simulink model "hybrid_discharge_sc_bat"  (R2014b)
settings: Solver=ode23t  StartTime=0.0  StopTime=10  RelTol=1e-3
undefined symbols (not defined in the file or in its folder): Hydride, Metal, Nickel
libraries: powerlib x9, simulink x3, electricdrivelib x2
settings Model: Creator=Administrator  LastModifiedBy=Administrator

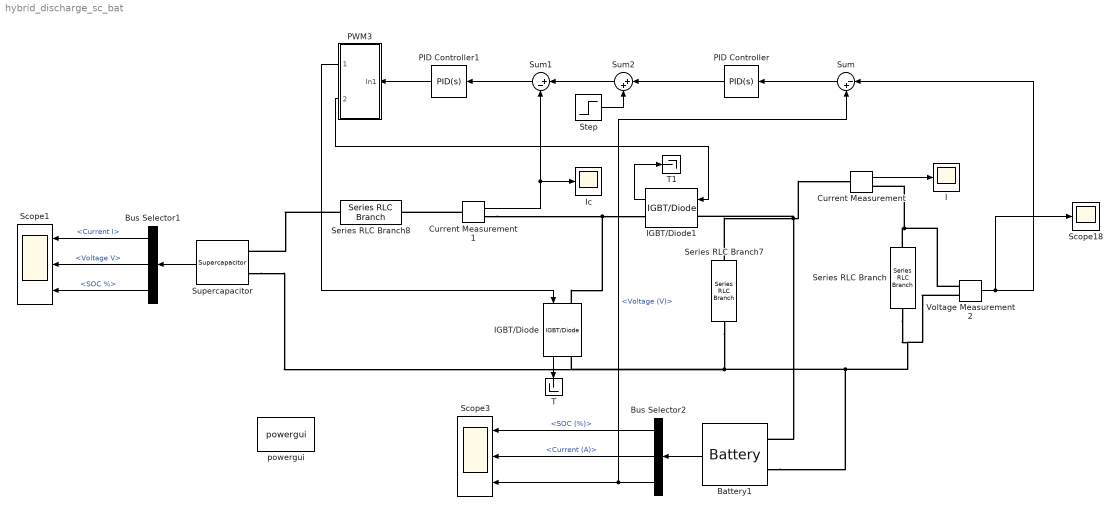
== system hybrid_discharge_sc_bat ==
  Battery1 : electricdrivelib/Extra Sources/Battery  BatType=Nickel-Metal-Hydride  ShowDetailedParameters=off  NomV=380  NomQ=100  SOC=80  PresetModel=on  MaxQ=107.6923  FullV=447.6271  Dis_rate=20  R=0.038  Normal_OP=96.1538  expZone="[412.2034            20]"  Dis_Char=off  current=[1.5 3]  Units=Ampere-hour  Batt_Tr=30
  Bus Selector1 : BusSelector  OutputSignals=Current I,Voltage V,SOC %
  Bus Selector2 : BusSelector  OutputSignals=SOC (%),Current (A),Voltage (V)
  Current Measurement : powerlib/Measurements/Current Measurement  PhasorSimulation=off  OutputType=Complex  PSBequivalent=0
  Current Measurement1 : powerlib/Measurements/Current Measurement  PhasorSimulation=off  OutputType=Complex  PSBequivalent=0
  I : Scope
      settings: YMin=750  YMax=1100  SaveName=ScopeData21  MaxDataPoints=5000000
  IGBT/Diode : powerlib/Power Electronics/IGBT//Diode  Ron=1e-3  Rs=1e5  Cs=inf  Measurements=on
  IGBT/Diode1 : powerlib/Power Electronics/IGBT//Diode  Ron=1e-3  Rs=1e5  Cs=inf  Measurements=on
  Ic : Scope
      settings: YMin=750  YMax=1100  SaveName=ScopeData3  MaxDataPoints=5000000
  PID Controller : simulink/Continuous/PID Controller  Controller=PID  TimeDomain=Continuous-time  SampleTime=-1  IntegratorMethod=Forward Euler  FilterMethod=Forward Euler  Form=Parallel  P=0.1  I=10  D=0  N=100  InitialConditionSource=internal  InitialConditionForIntegrator=0  InitialConditionForFilter=0  ExternalReset=none  LimitOutput=off  UpperSaturationLimit=inf  LowerSaturationLimit=-inf  LinearizeAsGain=on  AntiWindupMode=none  Kb=1  TrackingMode=off  Kt=1  PParamMin=[]  PParamMax=[]  IParamMin=[]  IParamMax=[]  DParamMin=[]  DParamMax=[]  NParamMin=[]  NParamMax=[]  KbParamMin=[]  KbParamMax=[]  KtParamMin=[]  KtParamMax=[]  POutMin=[]  POutMax=[]  IOutMin=[]  IOutMax=[]  DOutMin=[]  DOutMax=[]  NOutMin=[]  NOutMax=[]  KbOutMin=[]  KbOutMax=[]  KtOutMin=[]  KtOutMax=[]  IntegratorOutMin=[]  IntegratorOutMax=[]  FilterOutMin=[]  FilterOutMax=[]  SumOutMin=[]  SumOutMax=[]  SumI1OutMin=[]  SumI1OutMax=[]  SumI2OutMin=[]  SumI2OutMax=[]  SumI3OutMin=[]  SumI3OutMax=[]  SumDOutMin=[]  SumDOutMax=[]  SaturationOutMin=[]  SaturationOutMax=[]  IntegratorContinuousStateAttributes=''  IntegratorStateMustResolveToSignalObject=off  IntegratorRTWStateStorageClass=Auto  FilterContinuousStateAttributes=''  FilterStateMustResolveToSignalObject=off  FilterRTWStateStorageClass=Auto  DifferentiatorICPrevScaledInput=0  DifferentiatorOutMin=[]  DifferentiatorOutMax=[]  UseFilter=on
  PID Controller1 : simulink/Continuous/PID Controller  Controller=PID  TimeDomain=Continuous-time  SampleTime=-1  IntegratorMethod=Forward Euler  FilterMethod=Forward Euler  Form=Parallel  P=0.1  I=1  D=0  N=100  InitialConditionSource=internal  InitialConditionForIntegrator=0  InitialConditionForFilter=0  ExternalReset=none  LimitOutput=off  UpperSaturationLimit=inf  LowerSaturationLimit=-inf  LinearizeAsGain=on  AntiWindupMode=none  Kb=1  TrackingMode=off  Kt=1  PParamMin=[]  PParamMax=[]  IParamMin=[]  IParamMax=[]  DParamMin=[]  DParamMax=[]  NParamMin=[]  NParamMax=[]  KbParamMin=[]  KbParamMax=[]  KtParamMin=[]  KtParamMax=[]  POutMin=[]  POutMax=[]  IOutMin=[]  IOutMax=[]  DOutMin=[]  DOutMax=[]  NOutMin=[]  NOutMax=[]  KbOutMin=[]  KbOutMax=[]  KtOutMin=[]  KtOutMax=[]  IntegratorOutMin=[]  IntegratorOutMax=[]  FilterOutMin=[]  FilterOutMax=[]  SumOutMin=[]  SumOutMax=[]  SumI1OutMin=[]  SumI1OutMax=[]  SumI2OutMin=[]  SumI2OutMax=[]  SumI3OutMin=[]  SumI3OutMax=[]  SumDOutMin=[]  SumDOutMax=[]  SaturationOutMin=[]  SaturationOutMax=[]  IntegratorContinuousStateAttributes=''  IntegratorStateMustResolveToSignalObject=off  IntegratorRTWStateStorageClass=Auto  FilterContinuousStateAttributes=''  FilterStateMustResolveToSignalObject=off  FilterRTWStateStorageClass=Auto  DifferentiatorICPrevScaledInput=0  DifferentiatorOutMin=[]  DifferentiatorOutMax=[]  UseFilter=on
  PWM3 : Subsystem
  Scope1 : Scope  NumInputPorts=3
      settings: YMin=325~-5~-5  YMax=550~5~5
  Scope18 : Scope
      settings: TimeRange=1.5  YMin=378.7  YMax=379.225  SaveName=ScopeData23  MaxDataPoints=5000000
  Scope3 : Scope  NumInputPorts=3
      settings: YMin=325~0~-5  YMax=550~50~5  SaveName=ScopeData2
  Series RLC Branch : powerlib/Elements/Series RLC Branch  LConnTagsString=__new0  RConnTagsString=__new0  BranchType=R  Resistance=10  Inductance=1e-3  SetiL0=off  InitialCurrent=0  Capacitance=1e-6  Setx0=off  InitialVoltage=0  Measurements=None
  Series RLC Branch7 : powerlib/Elements/Series RLC Branch  LConnTagsString=__new0  RConnTagsString=__new0  BranchType=C  Resistance=1  Inductance=1e-3  SetiL0=off  InitialCurrent=0  Capacitance=45e-4  Setx0=off  InitialVoltage=0  Measurements=None
  Series RLC Branch8 : powerlib/Elements/Series RLC Branch  LConnTagsString=__new0  RConnTagsString=__new0  BranchType=L  Resistance=1  Inductance=17.5e-4  SetiL0=off  InitialCurrent=0  Capacitance=1e-6  Setx0=off  InitialVoltage=0  Measurements=None
  Step : Step  Time=10  After=50  SampleTime=0
  Sum : Sum  Inputs=|-+
  Sum1 : Sum  Inputs=|+-
  Sum2 : Sum  Inputs=|++
  Supercapacitor : electricdrivelib/Extra Sources/Supercapacitor  C=27.5  Rdc=2.1e-3  Voltage=300  Ns=122  Np=1  Vinit=300  Temp=25  PresetModel=off  EstParam=off  Nc=6  r=1.23e-9  epsilon=6.0208e-10  Ich=10  Vstern="[0.161  2.7  7.8]"  Self_dis=on  Ioc=10  Vself="[48  47.8  47.06  44.65]"  demandeplot=off  I=10.2  Units=sec  Vmax=230  If=5.2e-3  deltaV=0.3  alpha=0.3  sec=1988
  T : Terminator
  T1 : Terminator
  Voltage Measurement2 : powerlib/Measurements/Voltage Measurement  PhasorSimulation=off  OutputType=Complex  PSBequivalent=0
  powergui : powerlib/powergui  Priority=1  SimulationMode=Discrete  SolverType=Tustin  SampleTime=5e-5  frequency=60  SPID=off  DisableSnubberDevices=off  DisableRonSwitches=off  DisableVfSwitches=off  SwTol=0  DisplayEquations=off  Interpol=off  methode=off  Ts=0  frequencyindice=0  Pbase=100e6  ErrMax=1e-4  Iterations=50  UnitsV=kV  UnitsW=MW  FunctionMessages=off  echomessages=off  HookPort=off  EnableUseOfTLC=off  x0status=blocks  RestoreLinks=warning  ResistiveCurrentMeasurement=off  Frange=[0:2:500]  Ylog=off  Xlog=on  ShowGrid=off  save=off  variable=ZData  structure=0  ZoomFFT=off  StartTime=0.0  cycles=1  DisplayStyle=1  fundamental=60  FreqAxis=off  MaxFrequency=1000  frequencyindicesteady=1  RmsSteady=1  display=off
  wires:
  Voltage Measurement2/1 -> Scope18/1, Sum/1
  Sum/1 -> PID Controller/1
  PID Controller/1 -> Sum2/1
  PID Controller1/1 -> PWM3/1(In1)
  Current Measurement/1 -> I/1
  PWM3/1(Out1) -> IGBT/Diode/1
  PWM3/2(Out2) -> IGBT/Diode1/1
  Supercapacitor/1 -> Bus Selector1/1
  Bus Selector1/1 -> Scope1/1  "<Current I>"
  Bus Selector1/2 -> Scope1/2  "<Voltage V>"
  Bus Selector1/3 -> Scope1/3  "<SOC %>"
  Sum2/1 -> Sum1/1
  Sum1/1 -> PID Controller1/1
  IGBT/Diode/1 -> T/1
  IGBT/Diode1/1 -> T1/1
  Current Measurement1/1 -> Ic/1, Sum1/2
  Battery1/1 -> Bus Selector2/1
  Bus Selector2/1 -> Scope3/1  "<SOC (%)>"
  Bus Selector2/2 -> Scope3/2  "<Current (A)>"
  Bus Selector2/3 -> Scope3/3, Sum/2  "<Voltage (V)>"
  Step/1 -> Sum2/2
  connections:
  Series RLC Branch8/LConn1 -- Supercapacitor/LConn1
  IGBT/Diode/LConn1 -- Current Measurement1/RConn1 -- IGBT/Diode1/RConn1
  Series RLC Branch7/RConn1 -- Battery1/LConn2 -- Series RLC Branch/RConn1 -- Voltage Measurement2/LConn2 -- Supercapacitor/LConn2 -- IGBT/Diode/RConn1
  Voltage Measurement2/LConn1 -- Series RLC Branch/LConn1 -- Current Measurement/RConn1
  Current Measurement1/LConn1 -- Series RLC Branch8/RConn1
  IGBT/Diode1/LConn1 -- Series RLC Branch7/LConn1 -- Battery1/LConn1 -- Current Measurement/LConn1

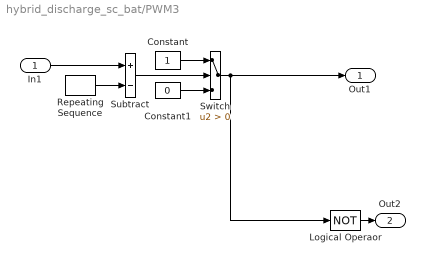
== system hybrid_discharge_sc_bat/PWM3 ==
  In1 : Inport
  Constant : Constant
  Constant1 : Constant  Value=0
  Logical Operaor : Logic  Operator=NOT  AllPortsSameDT=off  OutDataTypeStr=boolean
  Repeating Sequence : simulink/Sources/Repeating Sequence  rep_seq_t=[0 0.5e-4 1e-4]  rep_seq_y=[-1 1 -1]
  Subtract : Sum  Inputs=+-
  Switch : Switch  Criteria=u2 > Threshold
  Out1 : Outport
  Out2 : Outport  Port=2
  wires:
  Subtract/1 -> Switch/2
  Constant/1 -> Switch/1
  Constant1/1 -> Switch/3
  Switch/1 -> Out1/1, Logical Operaor/1
  In1/1 -> Subtract/1
  Repeating Sequence/1 -> Subtract/2
  Logical Operaor/1 -> Out2/1
